simulink model "RBDmodel_io"  (R2023a)
settings: Solver=ode15s  StartTime=0.0  StopTime=10  FixedStep=0.0001  RelTol=1e-3  AbsTol=1e-3  EnableMultiTasking=on
model workspace (MAT data in the model file):
  C_Gimbal_FIXED = 0.1
  C_IAP_FIXED = 0.01
  IAP_Pa = 0
  K_Gimbal_FIXED = 0
  K_IAP_FIXED = 0
  Left_EO = 0
  Left_IO = 0
  Left_MF = 0
  Left_RA = 0
  Moment_AR = 0
  Moment_FE = 7.5
  Moment_LB = 0
  Right_EO = 0
  Right_IO = 0
  Right_MF = 0
  Right_RA = 0
  a_FIXED = 1
  b_FIXED = 1
  muscle_color_FIXED = [0 0 1]
  muscle_radius_FIXED = 1
libraries: checkpacklib x3, simulink x1
(part 1 of 2)
settings Model: PacingRate=0.110000  Creator=Siril TD  LastModifiedBy=siril
settings SolverCC: ZeroCrossAlgorithm=Adaptive  AutoInsertRateTranBlk=on
settings DataIOCC: LimitDataPoints=on  MaxDataPoints=50000  ReturnWorkspaceOutputsName=SDOSimTest_Log
settings OptimizationCC: LifeSpan=inf
settings DebuggingCC: IgnoredZcDiagnostic=none  UnconnectedInputMsg=warning  UnconnectedOutputMsg=warning  UnconnectedLineMsg=warning  AllowSymbolicDim=off  SFUnexpectedBacktrackingDiag=warning  SFNoUnconditionalDefaultTransitionDiag=warning  SFExecutionAtInitializationDiag=none  ArithmeticOperatorsInVariantConditions=warning
settings ModelReferenceCC: EnableRefExpFcnMdlSchedulingChecks=on
settings SFSimCC: SimUseLocalCustomCode=off  CustomCodeUndefinedFunction=UseInterfaceOnly
settings RTWCC: RTWUseLocalCustomCode=off  DLArmComputeVersion=19.05
settings CodeAppCC: StateflowObjectComments=on
settings GRTTargetCC: TargetLangStandard=C89/C90 (ANSI)
settings ConfigComp: CovMetricSettings=dw  CovSaveCumulativeToWorkspaceVar=on  CovSaveSingleToWorkspaceVar=on  CovExternalEMLEnable=off  CovSFcnEnable=off
settings SimscapeCC: SimscapeLogSimulationStatistics=on  SimscapeLogDataHistory=10000

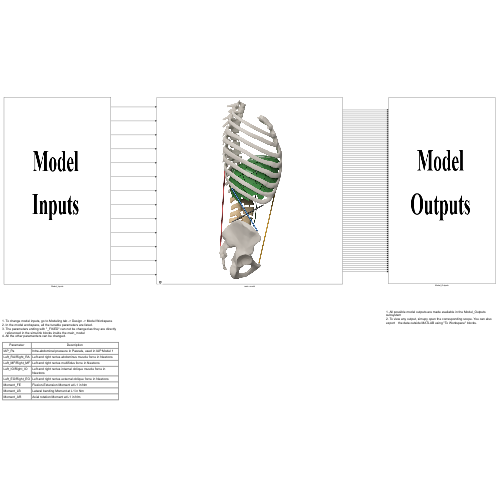
[thumbnail: Simulink's stored preview of the top-level diagram]
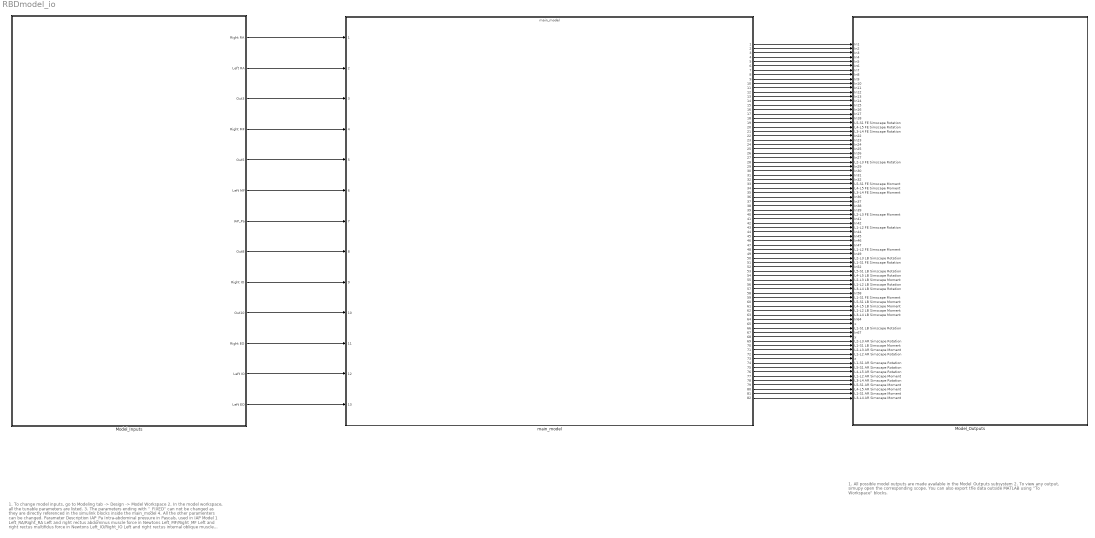
== system RBDmodel_io ==
  note: 1. All possible model outputs are made available in the Model_Outputs subsystem
      | 2. To view any output, simupy open the corresponding scope. You can also export the data outside MATLAB using "To Workspace" blocks.
  note: 1. To change model inputs, go to Modeling tab -> Design -> Model Workspace
      | 2. In the model workspace, all the tunable parameters are listed.
      | 3. The parameters ending with "_FIXED" can not be changed as they are directly
      | referenced in the simulink blocks inside the main_model
      | 4. All the other paramenters can be changed.
      |
      | Parameter
      | Description
      |
      | IAP_Pa
      | Intra-abdominal pressure in Pascals, used in IAP Model 1
      |
      | Left_RA/Right_RA
      | Left and right rectus abdominus muscle force in Newtons
      |
      | Left_MF/Right_MF
      | Left and right rectus multifidus force in Newtons
      |
      | Left_IO/Right_IO
      | Left and right rectus internal oblique muscle force in Newtons
      |
      | Left_EO/Right_EO
      | Left and right rectus external oblique force in Newtons
      |
      | Moment_FE
      | Flexion-Extension Moment at L1 in Nm
      |
      | Moment_LB
      | Lateral bending Moment at L1 in Nm
      |
      | Moment_AR
      | Axial rotation Moment at L1 in Nm
  Model_Inputs : Subsystem
      mask Display: image('$imagefile'); % Use "Edit Image" on toolstrip to change.
  Model_Outputs : Subsystem
      mask Display: image('$imagefile'); % Use "Edit Image" on toolstrip to change.
  main_model : ModelReference  ModelNameDialog=main_model  ModelReferenceVersion=6.157  CopyOfModelProtected=on
      mask Display: image('$imagefile'); % Use "Edit Image" on toolstrip to change.
  wires:
  Model_Inputs/1(Right RA) -> main_model/1
  Model_Inputs/2(Left RA) -> main_model/2
  Model_Inputs/3(Out3) -> main_model/3
  Model_Inputs/4(Right MF) -> main_model/4
  Model_Inputs/5(Out5) -> main_model/5
  Model_Inputs/6(Left MF) -> main_model/6
  Model_Inputs/7(IAP_Pa) -> main_model/7
  Model_Inputs/8(Out8) -> main_model/8
  Model_Inputs/9(Right IO) -> main_model/9
  Model_Inputs/10(Out10) -> main_model/10
  Model_Inputs/11(Right EO) -> main_model/11
  Model_Inputs/12(Left IO) -> main_model/12
  Model_Inputs/13(Left EO) -> main_model/13
  main_model/1 -> Model_Outputs/1(In1)
  main_model/2 -> Model_Outputs/2(In2)
  main_model/3 -> Model_Outputs/3(In3)
  main_model/4 -> Model_Outputs/4(In4)
  main_model/5 -> Model_Outputs/5(In5)
  main_model/6 -> Model_Outputs/6(In6)
  main_model/7 -> Model_Outputs/7(In7)
  main_model/8 -> Model_Outputs/8(In8)
  main_model/9 -> Model_Outputs/9(In9)
  main_model/10 -> Model_Outputs/10(In10)
  main_model/11 -> Model_Outputs/11(In11)
  main_model/12 -> Model_Outputs/12(In12)
  main_model/13 -> Model_Outputs/13(In13)
  main_model/14 -> Model_Outputs/14(In14)
  main_model/15 -> Model_Outputs/15(In15)
  main_model/16 -> Model_Outputs/16(In16)
  main_model/17 -> Model_Outputs/17(In17)
  main_model/18 -> Model_Outputs/18(In18)
  main_model/19 -> Model_Outputs/19(L5-S1 FE Simscape Rotation)
  main_model/20 -> Model_Outputs/20(L4-L5 FE Simscape Rotation)
  main_model/21 -> Model_Outputs/21(L3-L4 FE Simscape Rotation)
  main_model/22 -> Model_Outputs/22(In22)
  main_model/23 -> Model_Outputs/23(In23)
  main_model/24 -> Model_Outputs/24(In24)
  main_model/25 -> Model_Outputs/25(In25)
  main_model/26 -> Model_Outputs/26(In26)
  main_model/27 -> Model_Outputs/27(In27)
  main_model/28 -> Model_Outputs/28(L2-L3 FE Simscape Rotation)
  main_model/29 -> Model_Outputs/29(In29)
  main_model/30 -> Model_Outputs/30(In30)
  main_model/31 -> Model_Outputs/31(In31)
  main_model/32 -> Model_Outputs/32(In32)
  main_model/33 -> Model_Outputs/33(L5-S1 FE Simscape Moment)
  main_model/34 -> Model_Outputs/34(L4-L5 FE Simscape Moment)
  main_model/35 -> Model_Outputs/35(L3-L4 FE Simscape Moment)
  main_model/36 -> Model_Outputs/36(In36)
  main_model/37 -> Model_Outputs/37(In37)
  main_model/38 -> Model_Outputs/38(In38)
  main_model/39 -> Model_Outputs/39(In39)
  main_model/40 -> Model_Outputs/40(L2-L3 FE Simscape Moment)
  main_model/41 -> Model_Outputs/41(In41)
  main_model/42 -> Model_Outputs/42(In42)
  main_model/43 -> Model_Outputs/43(L1-L2 FE Simscape Rotation)
  main_model/44 -> Model_Outputs/44(In44)
  main_model/45 -> Model_Outputs/45(In45)
  main_model/46 -> Model_Outputs/46(In46)
  main_model/47 -> Model_Outputs/47(In47)
  main_model/48 -> Model_Outputs/48(L1-L2 FE Simscape Moment)
  main_model/49 -> Model_Outputs/49(In49)
  main_model/50 -> Model_Outputs/50(L2-L3 LB Simscape Rotation)
  main_model/51 -> Model_Outputs/51(L1-S1 FE Simscape Rotation)
  main_model/52 -> Model_Outputs/52(In52)
  main_model/53 -> Model_Outputs/53(L5-S1 LB Simscape Rotation)
  main_model/54 -> Model_Outputs/54(L4-L5 LB Simscape Rotation)
  main_model/55 -> Model_Outputs/55(L2-L3 LB Simscape Moment)
  main_model/56 -> Model_Outputs/56(L1-L2 LB Simscape Rotation)
  main_model/57 -> Model_Outputs/57(L3-L4 LB Simscape Rotation)
  main_model/58 -> Model_Outputs/58(In58)
  main_model/59 -> Model_Outputs/59(L1-S1 FE Simscape Moment)
  main_model/60 -> Model_Outputs/60(L5-S1 LB Simscape Moment)
  main_model/61 -> Model_Outputs/61(L4-L5 LB Simscape Moment)
  main_model/62 -> Model_Outputs/62(L1-L2 LB Simscape Moment)
  main_model/63 -> Model_Outputs/63(L3-L4 LB Simscape Moment)
  main_model/64 -> Model_Outputs/64(In64)
  main_model/65 -> Model_Outputs/65(x)
  main_model/66 -> Model_Outputs/66(L1-S1 LB Simscape Rotation)
  main_model/67 -> Model_Outputs/67(In67)
  main_model/68 -> Model_Outputs/68(y)
  main_model/69 -> Model_Outputs/69(L2-L3 AR Simscape Rotation)
  main_model/70 -> Model_Outputs/70(L1-S1 LB Simscape Moment)
  main_model/71 -> Model_Outputs/71(L2-L3 AR Simscape Moment)
  main_model/72 -> Model_Outputs/72(L1-L2 AR Simscape Rotation)
  main_model/73 -> Model_Outputs/73(z)
  main_model/74 -> Model_Outputs/74(L1-S1 AR Simscape Rotation)
  main_model/75 -> Model_Outputs/75(L5-S1 AR Simscape Rotation)
  main_model/76 -> Model_Outputs/76(L4-L5 AR Simscape Rotation)
  main_model/77 -> Model_Outputs/77(L1-L2 AR Simscape Moment)
  main_model/78 -> Model_Outputs/78(L3-L4 AR Simscape Rotation)
  main_model/79 -> Model_Outputs/79(L5-S1 AR Simscape Moment)
  main_model/80 -> Model_Outputs/80(L4-L5 AR Simscape Moment)
  main_model/81 -> Model_Outputs/81(L1-S1 AR Simscape Moment)
  main_model/82 -> Model_Outputs/82(L3-L4 AR Simscape Moment)

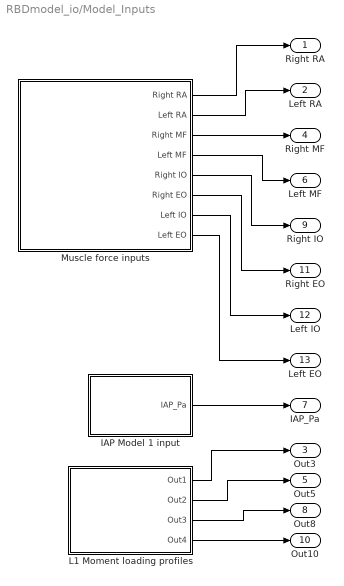
== system RBDmodel_io/Model_Inputs ==
  IAP Model 1 input : Subsystem
  L1 Moment loading profiles : Subsystem
  Muscle force inputs : Subsystem
  Right RA : Outport
  Left RA : Outport  Port=2
  Out3 : Outport  Port=3
  Right MF : Outport  Port=4
  Out5 : Outport  Port=5
  Left MF : Outport  Port=6
  IAP_Pa : Outport  Port=7
  Out8 : Outport  Port=8
  Right IO : Outport  Port=9
  Out10 : Outport  Port=10
  Right EO : Outport  Port=11
  Left IO : Outport  Port=12
  Left EO : Outport  Port=13
  wires:
  Muscle force inputs/4(Left MF) -> Left MF/1
  Muscle force inputs/8(Left EO) -> Left EO/1
  Muscle force inputs/3(Right MF) -> Right MF/1
  Muscle force inputs/7(Left IO) -> Left IO/1
  Muscle force inputs/2(Left RA) -> Left RA/1
  Muscle force inputs/6(Right EO) -> Right EO/1
  Muscle force inputs/1(Right RA) -> Right RA/1
  Muscle force inputs/5(Right IO) -> Right IO/1
  IAP Model 1 input/1(IAP_Pa) -> IAP_Pa/1
  L1 Moment loading profiles/1(Out1) -> Out3/1
  L1 Moment loading profiles/4(Out4) -> Out10/1
  L1 Moment loading profiles/3(Out3) -> Out8/1
  L1 Moment loading profiles/2(Out2) -> Out5/1

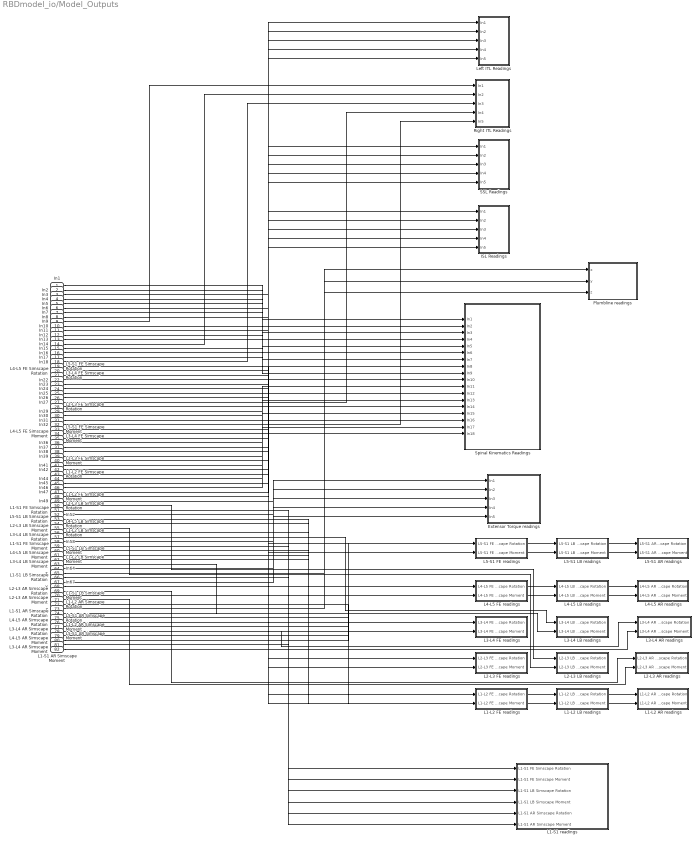
== system RBDmodel_io/Model_Outputs ==
  In1 : Inport
  In2 : Inport  Port=2
  In3 : Inport  Port=3
  In4 : Inport  Port=4
  In5 : Inport  Port=5
  In6 : Inport  Port=6
  In7 : Inport  Port=7
  In8 : Inport  Port=8
  In9 : Inport  Port=9
  In10 : Inport  Port=10
  In11 : Inport  Port=11
  In12 : Inport  Port=12
  In13 : Inport  Port=13
  In14 : Inport  Port=14
  In15 : Inport  Port=15
  In16 : Inport  Port=16
  In17 : Inport  Port=17
  In18 : Inport  Port=18
  L5-S1 FE Simscape Rotation : Inport  Port=19
  L4-L5 FE Simscape Rotation : Inport  Port=20
  L3-L4 FE Simscape Rotation : Inport  Port=21
  In22 : Inport  Port=22
  In23 : Inport  Port=23
  In24 : Inport  Port=24
  In25 : Inport  Port=25
  In26 : Inport  Port=26
  In27 : Inport  Port=27
  L2-L3 FE Simscape Rotation : Inport  Port=28
  In29 : Inport  Port=29
  In30 : Inport  Port=30
  In31 : Inport  Port=31
  In32 : Inport  Port=32
  L5-S1 FE Simscape Moment : Inport  Port=33
  L4-L5 FE Simscape Moment : Inport  Port=34
  L3-L4 FE Simscape Moment : Inport  Port=35
  In36 : Inport  Port=36
  In37 : Inport  Port=37
  In38 : Inport  Port=38
  In39 : Inport  Port=39
  L2-L3 FE Simscape Moment : Inport  Port=40
  In41 : Inport  Port=41
  In42 : Inport  Port=42
  L1-L2 FE Simscape Rotation : Inport  Port=43
  In44 : Inport  Port=44
  In45 : Inport  Port=45
  In46 : Inport  Port=46
  In47 : Inport  Port=47
  L1-L2 FE Simscape Moment : Inport  Port=48
  In49 : Inport  Port=49
  L2-L3 LB Simscape Rotation : Inport  Port=50
  L1-S1 FE Simscape Rotation : Inport  Port=51
  In52 : Inport  Port=52
  L5-S1 LB Simscape Rotation : Inport  Port=53
  L4-L5 LB Simscape Rotation : Inport  Port=54
  L2-L3 LB Simscape Moment : Inport  Port=55
  L1-L2 LB Simscape Rotation : Inport  Port=56
  L3-L4 LB Simscape Rotation : Inport  Port=57
  In58 : Inport  Port=58
  L1-S1 FE Simscape Moment : Inport  Port=59
  L5-S1 LB Simscape Moment : Inport  Port=60
  L4-L5 LB Simscape Moment : Inport  Port=61
  L1-L2 LB Simscape Moment : Inport  Port=62
  L3-L4 LB Simscape Moment : Inport  Port=63
  In64 : Inport  Port=64
  x : Inport  Port=65
  L1-S1 LB Simscape Rotation : Inport  Port=66
  In67 : Inport  Port=67
  y : Inport  Port=68
  L2-L3 AR Simscape Rotation : Inport  Port=69
  L1-S1 LB Simscape Moment : Inport  Port=70
  L2-L3 AR Simscape Moment : Inport  Port=71
  L1-L2 AR Simscape Rotation : Inport  Port=72
  z : Inport  Port=73
  L1-S1 AR Simscape Rotation : Inport  Port=74
  L5-S1 AR Simscape Rotation : Inport  Port=75
  L4-L5 AR Simscape Rotation : Inport  Port=76
  L1-L2 AR Simscape Moment : Inport  Port=77
  L3-L4 AR Simscape Rotation : Inport  Port=78
  L5-S1 AR Simscape Moment : Inport  Port=79
  L4-L5 AR Simscape Moment : Inport  Port=80
  L1-S1 AR Simscape Moment : Inport  Port=81
  L3-L4 AR Simscape Moment : Inport  Port=82
  Extensor Torque readings : Subsystem
  ISL Readings : Subsystem
  L1-L2 AR readings : Subsystem
  L1-L2 FE readings : Subsystem
  L1-L2 LB readings : Subsystem
  L1-S1 readings : Subsystem
  L2-L3 AR readings : Subsystem
  L2-L3 FE readings : Subsystem
  L2-L3 LB readings : Subsystem
  L3-L4 AR readings : Subsystem
  L3-L4 FE readings : Subsystem
  L3-L4 LB readings : Subsystem
  L4-L5 AR readings : Subsystem
  L4-L5 FE readings : Subsystem
  L4-L5 LB readings : Subsystem
  L5-S1 AR readings : Subsystem
  L5-S1 FE readings : Subsystem
  L5-S1 LB readings : Subsystem
  Left ITL Readings : Subsystem
  Plumbline readings : Subsystem
  Right ITL Readings : Subsystem
  SSL Readings : Subsystem
  Spinal Kinematics Readings : Subsystem
  wires:
  L1-L2 FE Simscape Rotation/1 -> L1-L2 FE readings/1(L1-L2 FE Simscape Rotation)
  L2-L3 LB Simscape Rotation/1 -> L2-L3 LB readings/1(L2-L3 LB Simscape Rotation)
  L1-S1 FE Simscape Rotation/1 -> L1-S1 readings/1(L1-S1 FE Simscape Rotation)
  In38/1 -> Left ITL Readings/4(In4)
  In8/1 -> Left ITL Readings/1(In1)
  In4/1 -> Spinal Kinematics Readings/3(In3)
  In49/1 -> Extensor Torque readings/1(In1)
  L3-L4 AR Simscape Moment/1 -> L3-L4 AR readings/2(L3-L4 AR Simscape Moment)
  In13/1 -> SSL Readings/2(In2)
  In17/1 -> Spinal Kinematics Readings/9(In9)
  In25/1 -> Spinal Kinematics Readings/11(In11)
  L1-S1 FE Simscape Moment/1 -> L1-S1 readings/2(L1-S1 FE Simscape Moment)
  L1-S1 AR Simscape Moment/1 -> L1-S1 readings/6(L1-S1 AR Simscape Moment)
  L5-S1 LB Simscape Moment/1 -> L5-S1 LB readings/2(L5-S1 LB Simscape Moment)
  L3-L4 AR Simscape Rotation/1 -> L3-L4 AR readings/1(L3-L4 AR Simscape Rotation)
  In58/1 -> Extensor Torque readings/3(In3)
  L1-L2 LB Simscape Moment/1 -> L1-L2 LB readings/2(L1-L2 LB Simscape Moment)
  L1-L2 LB Simscape Rotation/1 -> L1-L2 LB readings/1(L1-L2 LB Simscape Rotation)
  In16/1 -> Left ITL Readings/2(In2)
  L1-L2 FE Simscape Moment/1 -> L1-L2 FE readings/2(L1-L2 FE Simscape Moment)
  In42/1 -> SSL Readings/5(In5)
  In9/1 -> Right ITL Readings/1(In1)
  L5-S1 FE Simscape Moment/1 -> L5-S1 FE readings/2(L5-S1 FE Simscape Moment)
  L4-L5 FE Simscape Rotation/1 -> L4-L5 FE readings/1(L4-L5 FE Simscape Rotation)
  In36/1 -> Spinal Kinematics Readings/14(In14)
  In44/1 -> Spinal Kinematics Readings/17(In17)
  x/1 -> Plumbline readings/1(x)
  In26/1 -> Left ITL Readings/3(In3)
  L3-L4 FE Simscape Rotation/1 -> L3-L4 FE readings/1(L3-L4 FE Simscape Rotation)
  In7/1 -> Spinal Kinematics Readings/5(In5)
  In24/1 -> SSL Readings/3(In3)
  In15/1 -> Spinal Kinematics Readings/8(In8)
  In11/1 -> ISL Readings/2(In2)
  In18/1 -> Right ITL Readings/3(In3)
  L2-L3 AR Simscape Moment/1 -> L2-L3 AR readings/2(L2-L3 AR Simscape Moment)
  L5-S1 FE Simscape Rotation/1 -> L5-S1 FE readings/1(L5-S1 FE Simscape Rotation)
  In37/1 -> ISL Readings/4(In4)
  L1-L2 AR Simscape Moment/1 -> L1-L2 AR readings/2(L1-L2 AR Simscape Moment)
  In46/1 -> Spinal Kinematics Readings/18(In18)
  L5-S1 AR Simscape Moment/1 -> L5-S1 AR readings/2(L5-S1 AR Simscape Moment)
  In14/1 -> Right ITL Readings/2(In2)
  In3/1 -> ISL Readings/1(In1)
  In47/1 -> ISL Readings/5(In5)
  L5-S1 LB Simscape Rotation/1 -> L5-S1 LB readings/1(L5-S1 LB Simscape Rotation)
  In32/1 -> Right ITL Readings/5(In5)
  L5-S1 AR Simscape Rotation/1 -> L5-S1 AR readings/1(L5-S1 AR Simscape Rotation)
  In1/1 -> Spinal Kinematics Readings/1(In1)
  In23/1 -> ISL Readings/3(In3)
  In45/1 -> Left ITL Readings/5(In5)
  L3-L4 LB Simscape Rotation/1 -> L3-L4 LB readings/1(L3-L4 LB Simscape Rotation)
  In12/1 -> Spinal Kinematics Readings/7(In7)
  In5/1 -> Spinal Kinematics Readings/4(In4)
  L2-L3 FE Simscape Moment/1 -> L2-L3 FE readings/2(L2-L3 FE Simscape Moment)
  In39/1 -> Spinal Kinematics Readings/15(In15)
  L3-L4 LB Simscape Moment/1 -> L3-L4 LB readings/2(L3-L4 LB Simscape Moment)
  L3-L4 FE Simscape Moment/1 -> L3-L4 FE readings/2(L3-L4 FE Simscape Moment)
  In29/1 -> Spinal Kinematics Readings/12(In12)
  In41/1 -> Spinal Kinematics Readings/16(In16)
  In22/1 -> Spinal Kinematics Readings/10(In10)
  L4-L5 FE Simscape Moment/1 -> L4-L5 FE readings/2(L4-L5 FE Simscape Moment)
  L2-L3 FE Simscape Rotation/1 -> L2-L3 FE readings/1(L2-L3 FE Simscape Rotation)
  In64/1 -> Extensor Torque readings/4(In4)
  L4-L5 LB Simscape Rotation/1 -> L4-L5 LB readings/1(L4-L5 LB Simscape Rotation)
  In67/1 -> Extensor Torque readings/5(In5)
  In27/1 -> Right ITL Readings/4(In4)
  L1-S1 LB Simscape Moment/1 -> L1-S1 readings/4(L1-S1 LB Simscape Moment)
  L4-L5 LB Simscape Moment/1 -> L4-L5 LB readings/2(L4-L5 LB Simscape Moment)
  In31/1 -> SSL Readings/4(In4)
  In30/1 -> Spinal Kinematics Readings/13(In13)
  z/1 -> Plumbline readings/3(z)
  y/1 -> Plumbline readings/2(y)
  L1-S1 AR Simscape Rotation/1 -> L1-S1 readings/5(L1-S1 AR Simscape Rotation)
  L2-L3 AR Simscape Rotation/1 -> L2-L3 AR readings/1(L2-L3 AR Simscape Rotation)
  L4-L5 AR Simscape Rotation/1 -> L4-L5 AR readings/1(L4-L5 AR Simscape Rotation)
  L1-L2 AR Simscape Rotation/1 -> L1-L2 AR readings/1(L1-L2 AR Simscape Rotation)
  In6/1 -> SSL Readings/1(In1)
  In2/1 -> Spinal Kinematics Readings/2(In2)
  L4-L5 AR Simscape Moment/1 -> L4-L5 AR readings/2(L4-L5 AR Simscape Moment)
  L2-L3 LB Simscape Moment/1 -> L2-L3 LB readings/2(L2-L3 LB Simscape Moment)
  In10/1 -> Spinal Kinematics Readings/6(In6)
  In52/1 -> Extensor Torque readings/2(In2)
  L1-S1 LB Simscape Rotation/1 -> L1-S1 readings/3(L1-S1 LB Simscape Rotation)

== system RBDmodel_io/Model_Inputs/IAP Model 1 input ==
  Constant96 : Constant  Value=IAP_Pa
  IAP_Pa : Outport
  wires:
  Constant96/1 -> IAP_Pa/1

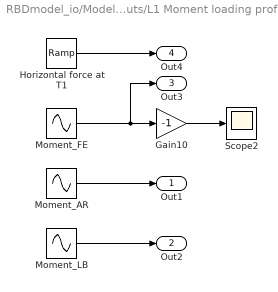
== system RBDmodel_io/Model_Inputs/L1 Moment loading profiles ==
  Gain10 : Gain  Gain=-1
  Horizontal force at T1 : simulink/Sources/Ramp  slope=0  start=0  InitialOutput=0
  Moment_AR : Sin  Amplitude=Moment_AR  SampleTime=0
  Moment_FE : Sin  Amplitude=-Moment_FE  SampleTime=0
  Moment_LB : Sin  Amplitude=-Moment_LB  SampleTime=0
  Scope2 : Scope
  Out1 : Outport
  Out2 : Outport  Port=2
  Out3 : Outport  Port=3
  Out4 : Outport  Port=4
  wires:
  Horizontal force at T1/1 -> Out4/1
  Moment_AR/1 -> Out1/1
  Moment_FE/1 -> Out3/1, Gain10/1
  Gain10/1 -> Scope2/1
  Moment_LB/1 -> Out2/1

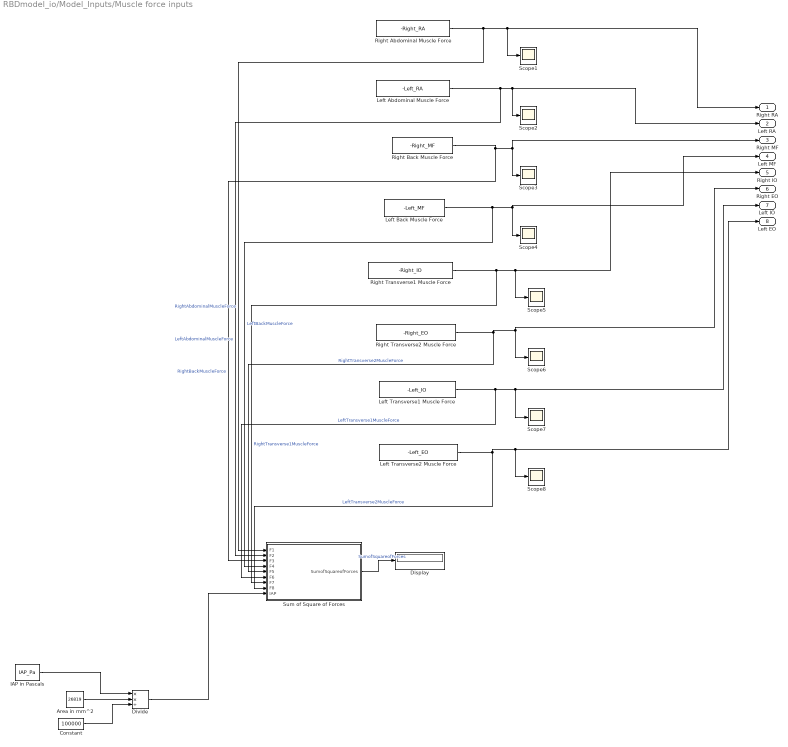
== system RBDmodel_io/Model_Inputs/Muscle force inputs ==
  Area in mm^2 : Constant  Value=26819
  Constant : Constant  Value=100000
  Display : Display
  Divide : Product  Inputs=**/
  IAP in Pascals : Constant  Value=IAP_Pa
  Left Abdominal Muscle Force : Constant  Value=-Left_RA
  Left Back Muscle Force : Constant  Value=-Left_MF
  Left Transverse1 Muscle Force : Constant  Value=-Left_IO
  Left Transverse2 Muscle Force : Constant  Value=-Left_EO
  Right Abdominal Muscle Force : Constant  Value=-Right_RA
  Right Back Muscle Force : Constant  Value=-Right_MF
  Right Transverse1 Muscle Force : Constant  Value=-Right_IO
  Right Transverse2 Muscle Force : Constant  Value=-Right_EO
  Scope{1..8} (8 alike) : Scope
  Sum of Square of Forces : MATLAB Function  TreatAsAtomicUnit=on
  Right RA : Outport
  Left RA : Outport  Port=2
  Right MF : Outport  Port=3
  Left MF : Outport  Port=4
  Right IO : Outport  Port=5
  Right EO : Outport  Port=6
  Left IO : Outport  Port=7
  Left EO : Outport  Port=8
  wires:
  Left Transverse2 Muscle Force/1 -> Left EO/1, Scope8/1, Sum of Square of Forces/8(F8)  "LeftTransverse2MuscleForce"
  Left Abdominal Muscle Force/1 -> Left RA/1, Scope2/1, Sum of Square of Forces/2(F2)  "LeftAbdominalMuscleForce"
  Sum of Square of Forces/1(SumofSquareofForces) -> Display/1  "SumofSquareofForces"
  Area in mm^2/1 -> Divide/2
  Left Back Muscle Force/1 -> Sum of Square of Forces/4(F4), Left MF/1, Scope4/1  "LeftBackMuscleForce"
  Divide/1 -> Sum of Square of Forces/9(IAP)
  Left Transverse1 Muscle Force/1 -> Left IO/1, Scope7/1, Sum of Square of Forces/6(F6)  "LeftTransverse1MuscleForce"
  Right Abdominal Muscle Force/1 -> Right RA/1, Scope1/1, Sum of Square of Forces/1(F1)  "RightAbdominalMuscleForce"
  Right Back Muscle Force/1 -> Right MF/1, Scope3/1, Sum of Square of Forces/3(F3)  "RightBackMuscleForce"
  Right Transverse2 Muscle Force/1 -> Right EO/1, Scope6/1, Sum of Square of Forces/5(F5)  "RightTransverse2MuscleForce"
  Right Transverse1 Muscle Force/1 -> Right IO/1, Scope5/1, Sum of Square of Forces/7(F7)  "RightTransverse1MuscleForce"
  IAP in Pascals/1 -> Divide/1
  Constant/1 -> Divide/3

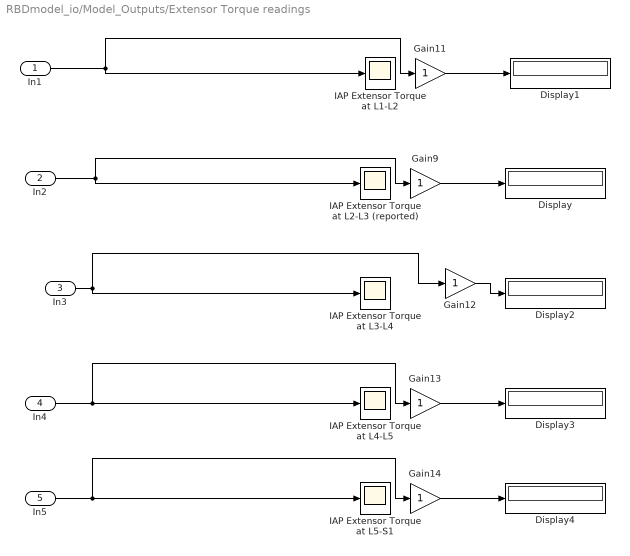
== system RBDmodel_io/Model_Outputs/Extensor Torque readings ==
  In1 : Inport
  In2 : Inport  Port=2
  In3 : Inport  Port=3
  In4 : Inport  Port=4
  In5 : Inport  Port=5
  Display{,1..4} (5 alike) : Display
      settings: Decimation=2
  Gain{9,11..14} (5 alike) : Gain
  IAP Extensor Torque at L1-L2 : Scope
  IAP Extensor Torque at L2-L3 (reported) : Scope
  IAP Extensor Torque at L3-L4 : Scope
  IAP Extensor Torque at L4-L5 : Scope
  IAP Extensor Torque at L5-S1 : Scope
  wires:
  Gain11/1 -> Display1/1
  Gain9/1 -> Display/1
  In5/1 -> Gain14/1, IAP Extensor Torque at L5-S1/1
  In2/1 -> Gain9/1, IAP Extensor Torque at L2-L3 (reported)/1
  Gain12/1 -> Display2/1
  In4/1 -> Gain13/1, IAP Extensor Torque at L4-L5/1
  In3/1 -> Gain12/1, IAP Extensor Torque at L3-L4/1
  Gain13/1 -> Display3/1
  In1/1 -> Gain11/1, IAP Extensor Torque at L1-L2/1
  Gain14/1 -> Display4/1

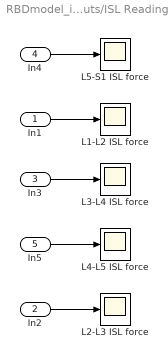
== system RBDmodel_io/Model_Outputs/ISL Readings ==
  In1 : Inport
  In2 : Inport  Port=2
  In3 : Inport  Port=3
  In4 : Inport  Port=4
  In5 : Inport  Port=5
  L1-L2 ISL force : Scope
  L2-L3 ISL force : Scope
  L3-L4 ISL force : Scope
  L4-L5 ISL force : Scope
  L5-S1 ISL force : Scope
  wires:
  In4/1 -> L5-S1 ISL force/1
  In2/1 -> L2-L3 ISL force/1
  In1/1 -> L1-L2 ISL force/1
  In3/1 -> L3-L4 ISL force/1
  In5/1 -> L4-L5 ISL force/1

== system RBDmodel_io/Model_Outputs/L1-L2 AR readings ==
  L1-L2 AR Simscape Rotation : Inport
  L1-L2 AR Simscape Moment : Inport  Port=2
  L1-L2 AR Moment : Scope
  L1-L2 AR Rotation : Scope
  L1-L2 AR Simscape : Record  FileSettingsInternal="{\"entries\":[{\"content\":{\"excelSettings\":{\"content\":{},\"type\":\"Streamout.ExcelSettings\"}},\"type\":\"Streamout.FileSettingStorage\",\"uuid\":\"559a99f2-f483-4c79-80a1-ce04f6e08210\"}],\"packageUris\":[\"http://schema.mathworks.com/mf0/streamout_blocks/R2020a\"],\"version\":\"1.0\"}"  Layout=[1 1]  SignalsInternal="{\"entries\":[{\"content\":{\"signals\":[{\"content\":{\"blockPath\":[\"RBDmodel_io/Model_Outputs/L1-L2 AR readings/L1-L2 AR Simscape\"],\"dimensions\":[1],\"domain\":\"RBDmodel_io/Model_Outputs/L1-L2 AR readings/L1-L2 AR Simscape\",\"lineColor\":\"#0072bd\",\"port\":1,\"sid\":[\"\"],\"signalID\":616,\"signalName\":\"L1-L2 AR Simscape Rotation\"},\"type\":\"RecordBlkView.Signal\",\"uuid\":\"a08438ad-5880-4f87-a807-1c5e94a78ca6\"},{\"content\":{\"blockPath\":[\"RBDmodel_io/Model_Outputs/L1-L2 AR readings/L1-L2 AR Simscape\"],\"dimensions\":[1],\"domain\":\"RBDmodel_io/Model_Outputs/L1-L2 AR readings/L1-L2 AR Simscape\",\"lineColor\":\"#d95319\",\"port\":2,\"sid\":[\"\"],\"signalID\":620,\"signalName\":\"L1-L2 AR Simscape Moment\"},\"type\":\"RecordBlkView.Signal\",\"uuid\":\"1f965d13-3b09-4b37-8057-c452996a0892\"}]},\"type\":\"RecordBlkView.InputSignals\",\"uuid\":\"455f967d-8ccc-4253-b99f-d7388e0f4159\"}],\"packageUris\":[\"http://schema.mathworks.com/mf0/streamout_blocks/R2020a\"],\"version\":\"1.0\"}"  VisualizationBindings="{\"xyplotplugin\":{\"info\":[{\"series\":[],\"subplotID\":1}]}}"  CompatibilityTag=XY
  wires:
  L1-L2 AR Simscape Rotation/1 -> L1-L2 AR Simscape/1, L1-L2 AR Rotation/1
  L1-L2 AR Simscape Moment/1 -> L1-L2 AR Simscape/2, L1-L2 AR Moment/1

== system RBDmodel_io/Model_Outputs/L1-L2 FE readings ==
  L1-L2 FE Simscape Rotation : Inport
  L1-L2 FE Simscape Moment : Inport  Port=2
  L1-L2 FE Moment : Scope
  L1-L2 FE Rotation : Scope
  L1-L2 FE Simscape : Record  FileSettingsInternal="{\"entries\":[{\"content\":{\"excelSettings\":{\"content\":{},\"type\":\"Streamout.ExcelSettings\"}},\"type\":\"Streamout.FileSettingStorage\",\"uuid\":\"f8c199f5-7adb-46eb-bc9a-f428016eea17\"}],\"packageUris\":[\"http://schema.mathworks.com/mf0/streamout_blocks/R2020a\"],\"version\":\"1.0\"}"  Layout=[1 1]  SignalsInternal="{\"entries\":[{\"content\":{\"signals\":[{\"content\":{\"blockPath\":[\"RBDmodel_io/Model_Outputs/L1-L2 FE readings/L1-L2 FE Simscape\"],\"dimensions\":[1],\"domain\":\"RBDmodel_io/Model_Outputs/L1-L2 FE readings/L1-L2 FE Simscape\",\"lineColor\":\"#a2142f\",\"port\":1,\"sid\":[\"\"],\"signalID\":528,\"signalName\":\"L1-L2 FE Simscape Rotation\"},\"type\":\"RecordBlkView.Signal\",\"uuid\":\"dc8ecc1e-03b5-4430-83df-60db4228367d\"},{\"content\":{\"blockPath\":[\"RBDmodel_io/Model_Outputs/L1-L2 FE readings/L1-L2 FE Simscape\"],\"dimensions\":[1],\"domain\":\"RBDmodel_io/Model_Outputs/L1-L2 FE readings/L1-L2 FE Simscape\",\"lineColor\":\"#139fff\",\"port\":2,\"sid\":[\"\"],\"signalID\":532,\"signalName\":\"L1-L2 FE Simscape Moment\"},\"type\":\"RecordBlkView.Signal\",\"uuid\":\"9260aa92-a1c0-44ed-9872-49de3e6ddb96\"}]},\"type\":\"RecordBlkView.InputSignals\",\"uuid\":\"bae95716-194d-4808-9340-0a920eae9afd\"}],\"packageUris\":[\"http://schema.mathworks.com/mf0/streamout_blocks/R2020a\"],\"version\":\"1.0\"}"  VisualizationBindings="{\"xyplotplugin\":{\"info\":[{\"series\":[],\"subplotID\":1}]}}"  CompatibilityTag=XY
  wires:
  L1-L2 FE Simscape Rotation/1 -> L1-L2 FE Simscape/1, L1-L2 FE Rotation/1
  L1-L2 FE Simscape Moment/1 -> L1-L2 FE Simscape/2, L1-L2 FE Moment/1

== system RBDmodel_io/Model_Outputs/L1-L2 LB readings ==
  L1-L2 LB Simscape Rotation : Inport
  L1-L2 LB Simscape Moment : Inport  Port=2
  L1-L2 LB Moment : Scope
  L1-L2 LB Rotation : Scope
  L1-L2 LB Simscape : Record  FileSettingsInternal="{\"entries\":[{\"content\":{\"excelSettings\":{\"content\":{},\"type\":\"Streamout.ExcelSettings\"}},\"type\":\"Streamout.FileSettingStorage\",\"uuid\":\"adfe9368-4326-4e5f-8eb9-72754077bfc9\"}],\"packageUris\":[\"http://schema.mathworks.com/mf0/streamout_blocks/R2020a\"],\"version\":\"1.0\"}"  Layout=[1 1]  SignalsInternal="{\"entries\":[{\"content\":{\"signals\":[{\"content\":{\"blockPath\":[\"RBDmodel_io/Model_Outputs/L1-L2 LB readings/L1-L2 LB Simscape\"],\"dimensions\":[1],\"domain\":\"RBDmodel_io/Model_Outputs/L1-L2 LB readings/L1-L2 LB Simscape\",\"lineColor\":\"#ff6929\",\"port\":1,\"sid\":[\"\"],\"signalID\":592,\"signalName\":\"L1-L2 LB Simscape Rotation\"},\"type\":\"RecordBlkView.Signal\",\"uuid\":\"f99aae56-7d27-4887-a173-11fd7f179eb9\"},{\"content\":{\"blockPath\":[\"RBDmodel_io/Model_Outputs/L1-L2 LB readings/L1-L2 LB Simscape\"],\"dimensions\":[1],\"domain\":\"RBDmodel_io/Model_Outputs/L1-L2 LB readings/L1-L2 LB Simscape\",\"lineColor\":\"#b746ff\",\"port\":2,\"sid\":[\"\"],\"signalID\":596,\"signalName\":\"L1-L2 LB Simscape Moment\"},\"type\":\"RecordBlkView.Signal\",\"uuid\":\"ee8d3d68-608e-42fb-8980-66d7cda9df91\"}]},\"type\":\"RecordBlkView.InputSignals\",\"uuid\":\"4689e526-3fab-4f29-86a4-a3ce82d16586\"}],\"packageUris\":[\"http://schema.mathworks.com/mf0/streamout_blocks/R2020a\"],\"version\":\"1.0\"}"  VisualizationBindings="{\"xyplotplugin\":{\"info\":[{\"series\":[],\"subplotID\":1}]}}"  CompatibilityTag=XY
  wires:
  L1-L2 LB Simscape Moment/1 -> L1-L2 LB Simscape/2, L1-L2 LB Moment/1
  L1-L2 LB Simscape Rotation/1 -> L1-L2 LB Simscape/1, L1-L2 LB Rotation/1

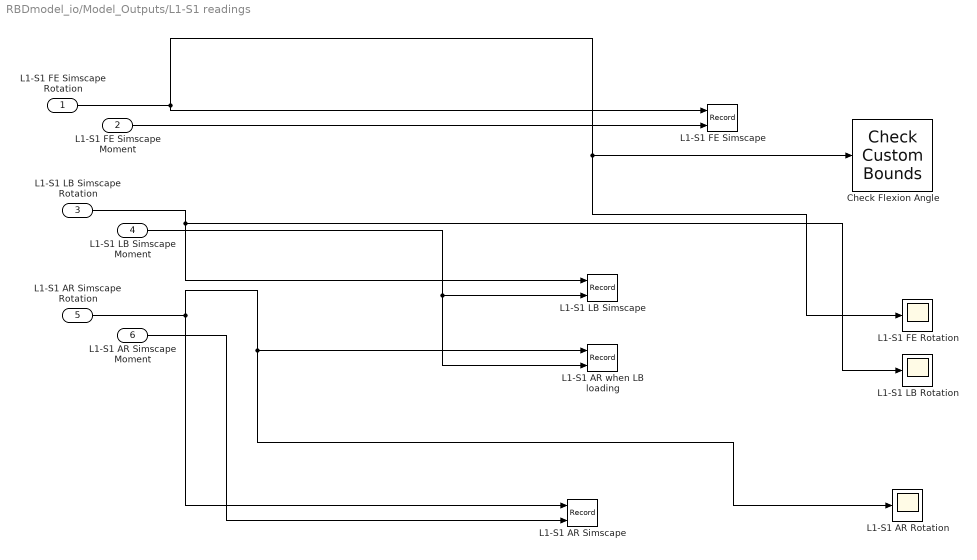
== system RBDmodel_io/Model_Outputs/L1-S1 readings ==
  L1-S1 FE Simscape Rotation : Inport
  L1-S1 FE Simscape Moment : Inport  Port=2
  L1-S1 LB Simscape Rotation : Inport  Port=3
  L1-S1 LB Simscape Moment : Inport  Port=4
  L1-S1 AR Simscape Rotation : Inport  Port=5
  L1-S1 AR Simscape Moment : Inport  Port=6
  Check Flexion Angle : checkpacklib/Check Custom Bounds  InstantiateOnLoad=on  enabled=off  stopWhenAssertionFail=off  export=off  ViewDlgPos=[100 200 510 390]  OpenViewOnLoad=off  LaunchViewOnOpen=off  TimeUnits=seconds  EnableUpperBound=on  UpperBoundTimes=[5 10]  UpperBoundAmplitudes=[51 51];  EnableLowerBound=on  LowerBoundTimes=[6 10]  LowerBoundAmplitudes=[49 49];
      settings: LibrarySourceBlock=sdolib/Signal Constraints/Check Custom Bounds
  L1-S1 AR Rotation : Scope
  L1-S1 AR Simscape : Record  FileSettingsInternal="{\"entries\":[{\"content\":{\"excelSettings\":{\"content\":{},\"type\":\"Streamout.ExcelSettings\"}},\"type\":\"Streamout.FileSettingStorage\",\"uuid\":\"942d7e30-9996-4677-ae83-8381080e1bc7\"}],\"packageUris\":[\"http://schema.mathworks.com/mf0/streamout_blocks/R2020a\"],\"version\":\"1.0\"}"  Layout=[1 1]  SignalsInternal="{\"entries\":[{\"content\":{\"signals\":[{\"content\":{\"blockPath\":[\"RBDmodel_io/Model_Outputs/L1-S1 readings/L1-S1 AR Simscape\"],\"dimensions\":[1,1],\"domain\":\"RBDmodel_io/Model_Outputs/L1-S1 readings/L1-S1 AR Simscape\",\"lineColor\":\"#fe330a\",\"port\":1,\"sid\":[\"\"],\"signalID\":552,\"signalName\":\"L1-S1 AR Simscape Rotation\"},\"type\":\"RecordBlkView.Signal\",\"uuid\":\"cc991e29-d1aa-490e-9d10-ccb8ee05ded1\"},{\"content\":{\"blockPath\":[\"RBDmodel_io/Model_Outputs/L1-S1 readings/L1-S1 AR Simscape\"],\"dimensions\":[1],\"domain\":\"RBDmodel_io/Model_Outputs/L1-S1 readings/L1-S1 AR Simscape\",\"lineColor\":\"#22b573\",\"port\":2,\"sid\":[\"\"],\"signalID\":556,\"signalName\":\"L1-S1 AR Simscape Moment\"},\"type\":\"RecordBlkView.Signal\",\"uuid\":\"f9e106c8-fd2a-469f-bcc0-818883d5f07c\"}]},\"type\":\"RecordBlkView.InputSignals\",\"uuid\":\"a8929c3a-9183-4609-a6d1-d4b66d45c2d8\"}],\"packageUris\":[\"http://schema.mathworks.com/mf0/streamout_blocks/R2020a\"],\"version\":\"1.0\"}"  VisualizationBindings="{\"xyplotplugin\":{\"info\":[{\"series\":[],\"subplotID\":1}]}}"  CompatibilityTag=XY
  L1-S1 AR when LB loading : Record  FileSettingsInternal="{\"entries\":[{\"content\":{\"excelSettings\":{\"content\":{},\"type\":\"Streamout.ExcelSettings\"}},\"type\":\"Streamout.FileSettingStorage\",\"uuid\":\"33f4ea06-4bd5-449a-8eae-33b928c149c0\"}],\"packageUris\":[\"http://schema.mathworks.com/mf0/streamout_blocks/R2020a\"],\"version\":\"1.0\"}"  Layout=[1 1]  SignalsInternal="{\"entries\":[{\"content\":{\"signals\":[{\"content\":{\"blockPath\":[\"RBDmodel_io/Model_Outputs/L1-S1 readings/L1-S1 AR when LB loading\"],\"dimensions\":[1,1],\"domain\":\"RBDmodel_io/Model_Outputs/L1-S1 readings/L1-S1 AR when LB loading\",\"lineColor\":\"#0072bd\",\"port\":1,\"sid\":[\"\"],\"signalID\":560,\"signalName\":\"L1-S1 AR Simscape Rotation\"},\"type\":\"RecordBlkView.Signal\",\"uuid\":\"bdb22080-7dd4-402b-8bfd-45777e76d01e\"},{\"content\":{\"blockPath\":[\"RBDmodel_io/Model_Outputs/L1-S1 readings/L1-S1 AR when LB loading\"],\"dimensions\":[1],\"domain\":\"RBDmodel_io/Model_Outputs/L1-S1 readings/L1-S1 AR when LB loading\",\"lineColor\":\"#d95319\",\"port\":2,\"sid\":[\"\"],\"signalID\":564,\"signalName\":\"L1-S1 LB Simscape Moment\"},\"type\":\"RecordBlkView.Signal\",\"uuid\":\"fb211177-e373-438c-a2d0-1ee4401105df\"}]},\"type\":\"RecordBlkView.InputSignals\",\"uuid\":\"bba3dc5a-d5b7-425b-9aaa-cbe82b1fca97\"}],\"packageUris\":[\"http://schema.mathworks.com/mf0/streamout_blocks/R2020a\"],\"version\":\"1.0\"}"  VisualizationBindings="{\"xyplotplugin\":{\"info\":[{\"series\":[],\"subplotID\":1}]}}"  CompatibilityTag=XY
  L1-S1 FE Rotation : Scope
  L1-S1 FE Simscape : Record  FileSettingsInternal="{\"entries\":[{\"content\":{\"excelSettings\":{\"content\":{},\"type\":\"Streamout.ExcelSettings\"}},\"type\":\"Streamout.FileSettingStorage\",\"uuid\":\"2716d3ce-848b-4703-a1db-63714f34e0d1\"}],\"packageUris\":[\"http://schema.mathworks.com/mf0/streamout_blocks/R2020a\"],\"version\":\"1.0\"}"  Layout=[1 1]  SignalsInternal="{\"entries\":[{\"content\":{\"signals\":[{\"content\":{\"blockPath\":[\"RBDmodel_io/Model_Outputs/L1-S1 readings/L1-S1 FE Simscape\"],\"dimensions\":[1,1],\"domain\":\"RBDmodel_io/Model_Outputs/L1-S1 readings/L1-S1 FE Simscape\",\"lineColor\":\"#ff6929\",\"plots\":[1],\"port\":1,\"sid\":[\"\"],\"signalID\":544,\"signalName\":\"L1-S1 FE Simscape Rotation\"},\"type\":\"RecordBlkView.Signal\",\"uuid\":\"5cfcc4a6-5d6d-4ac0-8b0c-8ff73ef6a195\"},{\"content\":{\"blockPath\":[\"RBDmodel_io/Model_Outputs/L1-S1 readings/L1-S1 FE Simscape\"],\"dimensions\":[1],\"domain\":\"RBDmodel_io/Model_Outputs/L1-S1 readings/L1-S1 FE Simscape\",\"lineColor\":\"#b746ff\",\"plots\":[1],\"port\":2,\"sid\":[\"\"],\"signalID\":548,\"signalName\":\"L1-S1 FE Simscape Moment\"},\"type\":\"RecordBlkView.Signal\",\"uuid\":\"51d8dc3d-842b-4676-be23-d846311d9746\"}]},\"type\":\"RecordBlkView.InputSignals\",\"uuid\":\"58dff127-f772-4e76-878c-6bd7d9beeb35\"}],\"packageUris\":[\"http://schema.mathworks.com/mf0/streamout_blocks/R2020a\"],\"version\":\"1.0\"}"  VisualizationBindings="{\"xyplotplugin\":{\"info\":[{\"series\":[{\"bindingParametersList\":[{\"parameter\":\"X-Axis\",\"signalID\":548,\"signalName\":\"L1-S1 FE Simscape Moment\"},{\"parameter\":\"Y-Axis\",\"signalID\":544,\"signalName\":\"L1-S1 FE Simscape Rotation\"}],\"seriesID\":39238}],\"subplotID\":1}]}}"  CompatibilityTag=XY
  L1-S1 LB Rotation : Scope
  L1-S1 LB Simscape : Record  FileSettingsInternal="{\"entries\":[{\"content\":{\"excelSettings\":{\"content\":{},\"type\":\"Streamout.ExcelSettings\"}},\"type\":\"Streamout.FileSettingStorage\",\"uuid\":\"5953cb44-6d2f-4aa3-829e-2fb388c55c97\"}],\"packageUris\":[\"http://schema.mathworks.com/mf0/streamout_blocks/R2020a\"],\"version\":\"1.0\"}"  Layout=[1 1]  SignalsInternal="{\"entries\":[{\"content\":{\"signals\":[{\"content\":{\"blockPath\":[\"RBDmodel_io/Model_Outputs/L1-S1 readings/L1-S1 LB Simscape\"],\"dimensions\":[1,1],\"domain\":\"RBDmodel_io/Model_Outputs/L1-S1 readings/L1-S1 LB Simscape\",\"lineColor\":\"#edb120\",\"port\":1,\"sid\":[\"\"],\"signalID\":568,\"signalName\":\"L1-S1 LB Simscape Rotation\"},\"type\":\"RecordBlkView.Signal\",\"uuid\":\"7bdad260-dcb3-443b-a084-0835adbd4350\"},{\"content\":{\"blockPath\":[\"RBDmodel_io/Model_Outputs/L1-S1 readings/L1-S1 LB Simscape\"],\"dimensions\":[1],\"domain\":\"RBDmodel_io/Model_Outputs/L1-S1 readings/L1-S1 LB Simscape\",\"lineColor\":\"#7e2f8e\",\"port\":2,\"sid\":[\"\"],\"signalID\":572,\"signalName\":\"L1-S1 LB Simscape Moment\"},\"type\":\"RecordBlkView.Signal\",\"uuid\":\"b70455e8-6f2e-4893-b1b2-86e8b8c6244d\"}]},\"type\":\"RecordBlkView.InputSignals\",\"uuid\":\"5a5a8b3c-c3c5-4984-b63f-288d87fb3552\"}],\"packageUris\":[\"http://schema.mathworks.com/mf0/streamout_blocks/R2020a\"],\"version\":\"1.0\"}"  VisualizationBindings="{\"xyplotplugin\":{\"info\":[{\"series\":[],\"subplotID\":1}]}}"  CompatibilityTag=XY
  wires:
  L1-S1 LB Simscape Rotation/1 -> L1-S1 LB Simscape/1, L1-S1 LB Rotation/1
  L1-S1 FE Simscape Rotation/1 -> Check Flexion Angle/1, L1-S1 FE Rotation/1, L1-S1 FE Simscape/1
  L1-S1 AR Simscape Rotation/1 -> L1-S1 AR when LB loading/1, L1-S1 AR Rotation/1, L1-S1 AR Simscape/1
  L1-S1 LB Simscape Moment/1 -> L1-S1 LB Simscape/2, L1-S1 AR when LB loading/2
  L1-S1 FE Simscape Moment/1 -> L1-S1 FE Simscape/2
  L1-S1 AR Simscape Moment/1 -> L1-S1 AR Simscape/2

== system RBDmodel_io/Model_Outputs/L2-L3 AR readings ==
  L2-L3 AR Simscape Rotation : Inport
  L2-L3 AR Simscape Moment : Inport  Port=2
  L2-L3 AR Moment : Scope
  L2-L3 AR Rotation : Scope
  L2-L3 AR Simscape : Record  FileSettingsInternal="{\"entries\":[{\"content\":{\"excelSettings\":{\"content\":{},\"type\":\"Streamout.ExcelSettings\"}},\"type\":\"Streamout.FileSettingStorage\",\"uuid\":\"804e996a-720c-429a-adbe-71c3c4fc65ab\"}],\"packageUris\":[\"http://schema.mathworks.com/mf0/streamout_blocks/R2020a\"],\"version\":\"1.0\"}"  Layout=[1 1]  SignalsInternal="{\"entries\":[{\"content\":{\"signals\":[{\"content\":{\"blockPath\":[\"RBDmodel_io/Model_Outputs/L2-L3 AR readings/L2-L3 AR Simscape\"],\"dimensions\":[1],\"domain\":\"RBDmodel_io/Model_Outputs/L2-L3 AR readings/L2-L3 AR Simscape\",\"lineColor\":\"#fe330a\",\"port\":1,\"sid\":[\"\"],\"signalID\":608,\"signalName\":\"L2-L3 AR Simscape Rotation\"},\"type\":\"RecordBlkView.Signal\",\"uuid\":\"1f84de15-4e49-4c42-9d61-d7de5e0626b0\"},{\"content\":{\"blockPath\":[\"RBDmodel_io/Model_Outputs/L2-L3 AR readings/L2-L3 AR Simscape\"],\"dimensions\":[1],\"domain\":\"RBDmodel_io/Model_Outputs/L2-L3 AR readings/L2-L3 AR Simscape\",\"lineColor\":\"#22b573\",\"port\":2,\"sid\":[\"\"],\"signalID\":612,\"signalName\":\"L2-L3 AR Simscape Moment\"},\"type\":\"RecordBlkView.Signal\",\"uuid\":\"d95f8373-04ff-4bc4-8774-a3aa9c3c0545\"}]},\"type\":\"RecordBlkView.InputSignals\",\"uuid\":\"3d60f1e9-dc61-4d3b-8745-b8fcfb86a502\"}],\"packageUris\":[\"http://schema.mathworks.com/mf0/streamout_blocks/R2020a\"],\"version\":\"1.0\"}"  VisualizationBindings="{\"xyplotplugin\":{\"info\":[{\"series\":[],\"subplotID\":1}]}}"  CompatibilityTag=XY
  wires:
  L2-L3 AR Simscape Rotation/1 -> L2-L3 AR Simscape/1, L2-L3 AR Rotation/1
  L2-L3 AR Simscape Moment/1 -> L2-L3 AR Simscape/2, L2-L3 AR Moment/1

== system RBDmodel_io/Model_Outputs/L2-L3 FE readings ==
  L2-L3 FE Simscape Rotation : Inport
  L2-L3 FE Simscape Moment : Inport  Port=2
  L2-L3 FE Moment : Scope
  L2-L3 FE Rotation : Scope
  L2-L3 FE Simscape : Record  FileSettingsInternal="{\"entries\":[{\"content\":{\"excelSettings\":{\"content\":{},\"type\":\"Streamout.ExcelSettings\"}},\"type\":\"Streamout.FileSettingStorage\",\"uuid\":\"89c04d1f-771b-4c87-96dc-ae8798b92010\"}],\"packageUris\":[\"http://schema.mathworks.com/mf0/streamout_blocks/R2020a\"],\"version\":\"1.0\"}"  Layout=[1 1]  SignalsInternal="{\"entries\":[{\"content\":{\"signals\":[{\"content\":{\"blockPath\":[\"RBDmodel_io/Model_Outputs/L2-L3 FE readings/L2-L3 FE Simscape\"],\"dimensions\":[1],\"domain\":\"RBDmodel_io/Model_Outputs/L2-L3 FE readings/L2-L3 FE Simscape\",\"lineColor\":\"#77ac30\",\"port\":1,\"sid\":[\"\"],\"signalID\":520,\"signalName\":\"L2-L3 FE Simscape Rotation\"},\"type\":\"RecordBlkView.Signal\",\"uuid\":\"34285638-c4b8-40df-8913-c52bbe534cf5\"},{\"content\":{\"blockPath\":[\"RBDmodel_io/Model_Outputs/L2-L3 FE readings/L2-L3 FE Simscape\"],\"dimensions\":[1],\"domain\":\"RBDmodel_io/Model_Outputs/L2-L3 FE readings/L2-L3 FE Simscape\",\"lineColor\":\"#4dbeee\",\"port\":2,\"sid\":[\"\"],\"signalID\":524,\"signalName\":\"L2-L3 FE Simscape Moment\"},\"type\":\"RecordBlkView.Signal\",\"uuid\":\"84c70ae9-48e5-436d-aa4f-b66209c9137d\"}]},\"type\":\"RecordBlkView.InputSignals\",\"uuid\":\"47dade43-6eb3-46ab-ba57-fcc5f4163f63\"}],\"packageUris\":[\"http://schema.mathworks.com/mf0/streamout_blocks/R2020a\"],\"version\":\"1.0\"}"  VisualizationBindings="{\"xyplotplugin\":{\"info\":[{\"series\":[],\"subplotID\":1}]}}"  CompatibilityTag=XY
  wires:
  L2-L3 FE Simscape Rotation/1 -> L2-L3 FE Simscape/1, L2-L3 FE Rotation/1
  L2-L3 FE Simscape Moment/1 -> L2-L3 FE Simscape/2, L2-L3 FE Moment/1

== system RBDmodel_io/Model_Outputs/L2-L3 LB readings ==
  L2-L3 LB Simscape Rotation : Inport
  L2-L3 LB Simscape Moment : Inport  Port=2
  L2-L3 LB Moment : Scope
  L2-L3 LB Rotation : Scope
  L2-L3 LB Simscape : Record  FileSettingsInternal="{\"entries\":[{\"content\":{\"excelSettings\":{\"content\":{},\"type\":\"Streamout.ExcelSettings\"}},\"type\":\"Streamout.FileSettingStorage\",\"uuid\":\"5336eb51-5057-4f95-8bb2-7bdb56d9221e\"}],\"packageUris\":[\"http://schema.mathworks.com/mf0/streamout_blocks/R2020a\"],\"version\":\"1.0\"}"  Layout=[1 1]  SignalsInternal="{\"entries\":[{\"content\":{\"signals\":[{\"content\":{\"blockPath\":[\"RBDmodel_io/Model_Outputs/L2-L3 LB readings/L2-L3 LB Simscape\"],\"dimensions\":[1],\"domain\":\"RBDmodel_io/Model_Outputs/L2-L3 LB readings/L2-L3 LB Simscape\",\"lineColor\":\"#ff6929\",\"port\":1,\"sid\":[\"\"],\"signalID\":536,\"signalName\":\"L2-L3 LB Simscape Rotation\"},\"type\":\"RecordBlkView.Signal\",\"uuid\":\"6afbef7c-623a-4fe9-bc4e-a0a4d48ba7d9\"},{\"content\":{\"blockPath\":[\"RBDmodel_io/Model_Outputs/L2-L3 LB readings/L2-L3 LB Simscape\"],\"dimensions\":[1],\"domain\":\"RBDmodel_io/Model_Outputs/L2-L3 LB readings/L2-L3 LB Simscape\",\"lineColor\":\"#b746ff\",\"port\":2,\"sid\":[\"\"],\"signalID\":540,\"signalName\":\"L2-L3 LB Simscape Moment\"},\"type\":\"RecordBlkView.Signal\",\"uuid\":\"6a8d8faa-cc53-47f3-96b2-bd242c0502d9\"}]},\"type\":\"RecordBlkView.InputSignals\",\"uuid\":\"3b9a9d84-ac03-49ca-b9b2-6faba7198416\"}],\"packageUris\":[\"http://schema.mathworks.com/mf0/streamout_blocks/R2020a\"],\"version\":\"1.0\"}"  VisualizationBindings="{\"xyplotplugin\":{\"info\":[{\"series\":[],\"subplotID\":1}]}}"  CompatibilityTag=XY
  wires:
  L2-L3 LB Simscape Rotation/1 -> L2-L3 LB Simscape/1, L2-L3 LB Rotation/1
  L2-L3 LB Simscape Moment/1 -> L2-L3 LB Simscape/2, L2-L3 LB Moment/1

== system RBDmodel_io/Model_Outputs/L3-L4 AR readings ==
  L3-L4 AR Simscape Rotation : Inport
  L3-L4 AR Simscape Moment : Inport  Port=2
  L3-L4 AR Moment : Scope
  L3-L4 AR Rotation : Scope
  L3-L4 AR Simscape : Record  FileSettingsInternal="{\"entries\":[{\"content\":{\"excelSettings\":{\"content\":{},\"type\":\"Streamout.ExcelSettings\"}},\"type\":\"Streamout.FileSettingStorage\",\"uuid\":\"c6647d97-1ed9-4e26-bfd8-8504da9e7b47\"}],\"packageUris\":[\"http://schema.mathworks.com/mf0/streamout_blocks/R2020a\"],\"version\":\"1.0\"}"  Layout=[1 1]  SignalsInternal="{\"entries\":[{\"content\":{\"signals\":[{\"content\":{\"blockPath\":[\"RBDmodel_io/Model_Outputs/L3-L4 AR readings/L3-L4 AR Simscape\"],\"dimensions\":[1],\"domain\":\"RBDmodel_io/Model_Outputs/L3-L4 AR readings/L3-L4 AR Simscape\",\"lineColor\":\"#a2142f\",\"port\":1,\"sid\":[\"\"],\"signalID\":640,\"signalName\":\"L3-L4 AR Simscape Rotation\"},\"type\":\"RecordBlkView.Signal\",\"uuid\":\"88cb88ae-0c3b-45cc-b0eb-addf378fcc9b\"},{\"content\":{\"blockPath\":[\"RBDmodel_io/Model_Outputs/L3-L4 AR readings/L3-L4 AR Simscape\"],\"dimensions\":[1],\"domain\":\"RBDmodel_io/Model_Outputs/L3-L4 AR readings/L3-L4 AR Simscape\",\"lineColor\":\"#139fff\",\"port\":2,\"sid\":[\"\"],\"signalID\":644,\"signalName\":\"L3-L4 AR Simscape Moment\"},\"type\":\"RecordBlkView.Signal\",\"uuid\":\"a499311d-e3fb-4884-85a6-6693f2c600cc\"}]},\"type\":\"RecordBlkView.InputSignals\",\"uuid\":\"1f9e1989-0ed7-4a80-9a86-98c9a38c21c5\"}],\"packageUris\":[\"http://schema.mathworks.com/mf0/streamout_blocks/R2020a\"],\"version\":\"1.0\"}"  VisualizationBindings="{\"xyplotplugin\":{\"info\":[{\"series\":[],\"subplotID\":1}]}}"  CompatibilityTag=XY
  wires:
  L3-L4 AR Simscape Rotation/1 -> L3-L4 AR Simscape/1, L3-L4 AR Rotation/1
  L3-L4 AR Simscape Moment/1 -> L3-L4 AR Simscape/2, L3-L4 AR Moment/1

== system RBDmodel_io/Model_Outputs/L3-L4 FE readings ==
  L3-L4 FE Simscape Rotation : Inport
  L3-L4 FE Simscape Moment : Inport  Port=2
  L3-L4 FE Moment : Scope
  L3-L4 FE Rotation : Scope
  L3-L4 FE Simscape : Record  FileSettingsInternal="{\"entries\":[{\"content\":{\"excelSettings\":{\"content\":{},\"type\":\"Streamout.ExcelSettings\"}},\"type\":\"Streamout.FileSettingStorage\",\"uuid\":\"6e997c07-ebd7-4601-b8a0-49771748ce3f\"}],\"packageUris\":[\"http://schema.mathworks.com/mf0/streamout_blocks/R2020a\"],\"version\":\"1.0\"}"  Layout=[1 1]  SignalsInternal="{\"entries\":[{\"content\":{\"signals\":[{\"content\":{\"blockPath\":[\"RBDmodel_io/Model_Outputs/L3-L4 FE readings/L3-L4 FE Simscape\"],\"dimensions\":[1],\"domain\":\"RBDmodel_io/Model_Outputs/L3-L4 FE readings/L3-L4 FE Simscape\",\"lineColor\":\"#edb120\",\"port\":1,\"sid\":[\"\"],\"signalID\":512,\"signalName\":\"L3-L4 FE Simscape Rotation\"},\"type\":\"RecordBlkView.Signal\",\"uuid\":\"49e4668a-08ce-42b7-b490-3a18e234e9ec\"},{\"content\":{\"blockPath\":[\"RBDmodel_io/Model_Outputs/L3-L4 FE readings/L3-L4 FE Simscape\"],\"dimensions\":[1],\"domain\":\"RBDmodel_io/Model_Outputs/L3-L4 FE readings/L3-L4 FE Simscape\",\"lineColor\":\"#7e2f8e\",\"port\":2,\"sid\":[\"\"],\"signalID\":516,\"signalName\":\"L3-L4 FE Simscape Moment\"},\"type\":\"RecordBlkView.Signal\",\"uuid\":\"a522955e-4152-4866-8e4d-94a6e28a0435\"}]},\"type\":\"RecordBlkView.InputSignals\",\"uuid\":\"cf5e947e-deb6-4535-b568-ca7916fe435d\"}],\"packageUris\":[\"http://schema.mathworks.com/mf0/streamout_blocks/R2020a\"],\"version\":\"1.0\"}"  VisualizationBindings="{\"xyplotplugin\":{\"info\":[{\"series\":[],\"subplotID\":1}]}}"  CompatibilityTag=XY
  wires:
  L3-L4 FE Simscape Rotation/1 -> L3-L4 FE Simscape/1, L3-L4 FE Rotation/1
  L3-L4 FE Simscape Moment/1 -> L3-L4 FE Simscape/2, L3-L4 FE Moment/1

== system RBDmodel_io/Model_Outputs/L3-L4 LB readings ==
  L3-L4 LB Simscape Rotation : Inport
  L3-L4 LB Simscape Moment : Inport  Port=2
  L3-L4 LB Moment : Scope
  L3-L4 LB Rotation : Scope
  L3-L4 LB Simscape : Record  FileSettingsInternal="{\"entries\":[{\"content\":{\"excelSettings\":{\"content\":{},\"type\":\"Streamout.ExcelSettings\"}},\"type\":\"Streamout.FileSettingStorage\",\"uuid\":\"561df458-1f99-4a26-95dd-1314aab399c8\"}],\"packageUris\":[\"http://schema.mathworks.com/mf0/streamout_blocks/R2020a\"],\"version\":\"1.0\"}"  Layout=[1 1]  SignalsInternal="{\"entries\":[{\"content\":{\"signals\":[{\"content\":{\"blockPath\":[\"RBDmodel_io/Model_Outputs/L3-L4 LB readings/L3-L4 LB Simscape\"],\"dimensions\":[1],\"domain\":\"RBDmodel_io/Model_Outputs/L3-L4 LB readings/L3-L4 LB Simscape\",\"lineColor\":\"#64d413\",\"port\":1,\"sid\":[\"\"],\"signalID\":600,\"signalName\":\"L3-L4 LB Simscape Rotation\"},\"type\":\"RecordBlkView.Signal\",\"uuid\":\"8317c680-519f-4af8-8421-bf95d386bf6c\"},{\"content\":{\"blockPath\":[\"RBDmodel_io/Model_Outputs/L3-L4 LB readings/L3-L4 LB Simscape\"],\"dimensions\":[1],\"domain\":\"RBDmodel_io/Model_Outputs/L3-L4 LB readings/L3-L4 LB Simscape\",\"lineColor\":\"#ff13a6\",\"port\":2,\"sid\":[\"\"],\"signalID\":604,\"signalName\":\"L3-L4 LB Simscape Moment\"},\"type\":\"RecordBlkView.Signal\",\"uuid\":\"9ecb05f8-6efe-47a6-95a2-91c67eef6695\"}]},\"type\":\"RecordBlkView.InputSignals\",\"uuid\":\"8cc82957-a579-427c-af2d-62607635289e\"}],\"packageUris\":[\"http://schema.mathworks.com/mf0/streamout_blocks/R2020a\"],\"version\":\"1.0\"}"  VisualizationBindings="{\"xyplotplugin\":{\"info\":[{\"series\":[],\"subplotID\":1}]}}"  CompatibilityTag=XY
  wires:
  L3-L4 LB Simscape Rotation/1 -> L3-L4 LB Simscape/1, L3-L4 LB Rotation/1
  L3-L4 LB Simscape Moment/1 -> L3-L4 LB Simscape/2, L3-L4 LB Moment/1

== system RBDmodel_io/Model_Outputs/L4-L5 AR readings ==
  L4-L5 AR Simscape Rotation : Inport
  L4-L5 AR Simscape Moment : Inport  Port=2
  L4-L5 AR Moment : Scope
  L4-L5 AR Rotation : Scope
  L4-L5 AR Simscape : Record  FileSettingsInternal="{\"entries\":[{\"content\":{\"excelSettings\":{\"content\":{},\"type\":\"Streamout.ExcelSettings\"}},\"type\":\"Streamout.FileSettingStorage\",\"uuid\":\"448f74a2-b9bb-42a4-93c9-cd0befa1b004\"}],\"packageUris\":[\"http://schema.mathworks.com/mf0/streamout_blocks/R2020a\"],\"version\":\"1.0\"}"  Layout=[1 1]  SignalsInternal="{\"entries\":[{\"content\":{\"signals\":[{\"content\":{\"blockPath\":[\"RBDmodel_io/Model_Outputs/L4-L5 AR readings/L4-L5 AR Simscape\"],\"dimensions\":[1],\"domain\":\"RBDmodel_io/Model_Outputs/L4-L5 AR readings/L4-L5 AR Simscape\",\"lineColor\":\"#77ac30\",\"port\":1,\"sid\":[\"\"],\"signalID\":632,\"signalName\":\"L4-L5 AR Simscape Rotation\"},\"type\":\"RecordBlkView.Signal\",\"uuid\":\"fedd6558-925e-4562-b1f0-a5a86250fe88\"},{\"content\":{\"blockPath\":[\"RBDmodel_io/Model_Outputs/L4-L5 AR readings/L4-L5 AR Simscape\"],\"dimensions\":[1],\"domain\":\"RBDmodel_io/Model_Outputs/L4-L5 AR readings/L4-L5 AR Simscape\",\"lineColor\":\"#4dbeee\",\"port\":2,\"sid\":[\"\"],\"signalID\":636,\"signalName\":\"L4-L5 AR Simscape Moment\"},\"type\":\"RecordBlkView.Signal\",\"uuid\":\"67a2ea15-be64-4c25-bd88-ee0bdd5a3fca\"}]},\"type\":\"RecordBlkView.InputSignals\",\"uuid\":\"9ea57243-aaf1-4206-a6be-cd4b424fd25d\"}],\"packageUris\":[\"http://schema.mathworks.com/mf0/streamout_blocks/R2020a\"],\"version\":\"1.0\"}"  VisualizationBindings="{\"xyplotplugin\":{\"info\":[{\"series\":[],\"subplotID\":1}]}}"  CompatibilityTag=XY
  wires:
  L4-L5 AR Simscape Moment/1 -> L4-L5 AR Simscape/2, L4-L5 AR Moment/1
  L4-L5 AR Simscape Rotation/1 -> L4-L5 AR Simscape/1, L4-L5 AR Rotation/1

== system RBDmodel_io/Model_Outputs/L4-L5 FE readings ==
  L4-L5 FE Simscape Rotation : Inport
  L4-L5 FE Simscape Moment : Inport  Port=2
  L4-L5 FE Moment : Scope
  L4-L5 FE Rotation : Scope
  L4-L5 FE Simscape : Record  FileSettingsInternal="{\"entries\":[{\"content\":{\"excelSettings\":{\"content\":{},\"type\":\"Streamout.ExcelSettings\"}},\"type\":\"Streamout.FileSettingStorage\",\"uuid\":\"fe75c6d0-7a4f-4a04-b453-1f931ebb75e4\"}],\"packageUris\":[\"http://schema.mathworks.com/mf0/streamout_blocks/R2020a\"],\"version\":\"1.0\"}"  Layout=[1 1]  SignalsInternal="{\"entries\":[{\"content\":{\"signals\":[{\"content\":{\"blockPath\":[\"RBDmodel_io/Model_Outputs/L4-L5 FE readings/L4-L5 FE Simscape\"],\"dimensions\":[1],\"domain\":\"RBDmodel_io/Model_Outputs/L4-L5 FE readings/L4-L5 FE Simscape\",\"lineColor\":\"#0072bd\",\"port\":1,\"sid\":[\"\"],\"signalID\":504,\"signalName\":\"L4-L5 FE Simscape Rotation\"},\"type\":\"RecordBlkView.Signal\",\"uuid\":\"58c5bf8e-9869-4d13-9760-2a13412a220e\"},{\"content\":{\"blockPath\":[\"RBDmodel_io/Model_Outputs/L4-L5 FE readings/L4-L5 FE Simscape\"],\"dimensions\":[1],\"domain\":\"RBDmodel_io/Model_Outputs/L4-L5 FE readings/L4-L5 FE Simscape\",\"lineColor\":\"#d95319\",\"port\":2,\"sid\":[\"\"],\"signalID\":508,\"signalName\":\"L4-L5 FE Simscape Moment\"},\"type\":\"RecordBlkView.Signal\",\"uuid\":\"c301fdec-abaa-4448-97e2-13ba1ae1987c\"}]},\"type\":\"RecordBlkView.InputSignals\",\"uuid\":\"87295ffe-a5a4-4932-89d2-68179a511438\"}],\"packageUris\":[\"http://schema.mathworks.com/mf0/streamout_blocks/R2020a\"],\"version\":\"1.0\"}"  VisualizationBindings="{\"xyplotplugin\":{\"info\":[{\"series\":[],\"subplotID\":1}]}}"  CompatibilityTag=XY
  wires:
  L4-L5 FE Simscape Rotation/1 -> L4-L5 FE Simscape/1, L4-L5 FE Rotation/1
  L4-L5 FE Simscape Moment/1 -> L4-L5 FE Simscape/2, L4-L5 FE Moment/1
